simulink model "S_SSM"  (R2022b)
settings: Solver=VariableStepAuto  StartTime=0.0  StopTime=20  RelTol=1e-3
values from neighbouring files (symbols this model uses):
  Kd = place(Ad,Bd,p_discretos)    [Sist_ident.m]
  Kdl = place(A,B,pc)    [Sist_ident.m]
  wnc = 4.6/(tsc*zitac)    [Sist_ident.m]
  zitac = sqrt(((log(Mpc))^2)/(((log(Mpc))^2)+ pi^2))    [Sist_ident.m]
undefined symbols (not defined in the file or in its folder): Ad, Adl, Bd, Bdl, Cd, Cdl
libraries: slpidlib x1
settings Model: Creator=juand  LastModifiedBy=juand

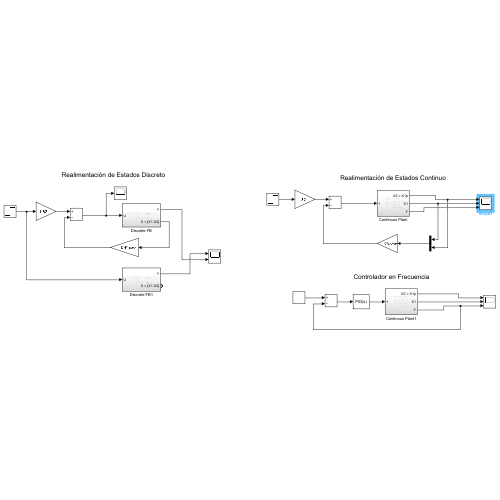
[thumbnail: Simulink's stored preview of the top-level diagram]
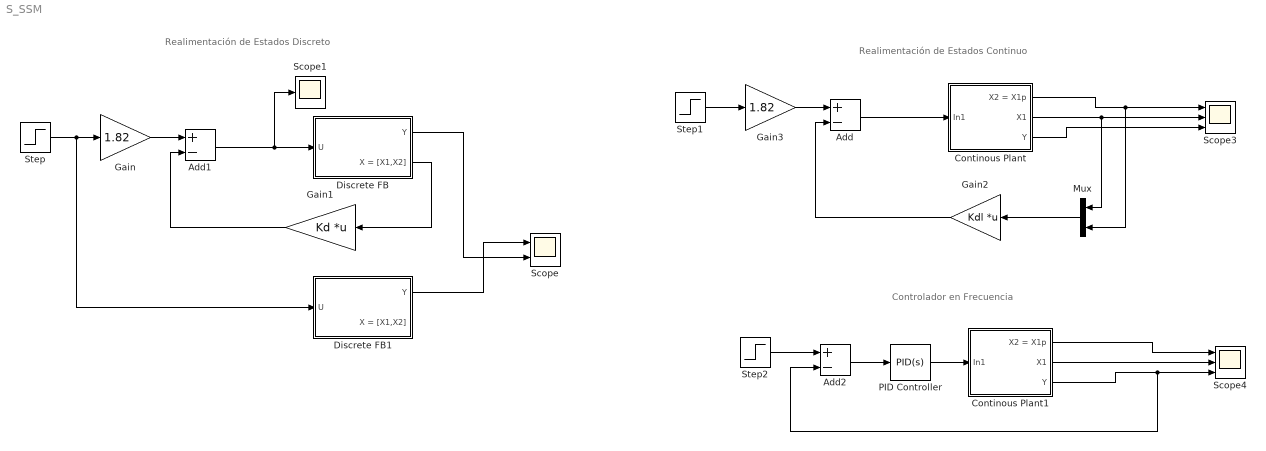
== system S_SSM ==
  note: Controlador en Frecuencia
  note: Realimentación de Estados Continuo
  note: Realimentación de Estados Discreto
  Add : Sum  Inputs=+-
  Add1 : Sum  Inputs=+-
  Add2 : Sum  Inputs=+-
  Continous Plant : Subsystem
  Continous Plant1 : Subsystem
  Discrete FB : Subsystem
  Discrete FB1 : Subsystem
  Gain : Gain  Gain=1.82
  Gain1 : Gain  Gain=Kd  Multiplication=Matrix(K*u) (u vector)
  Gain2 : Gain  Gain=Kdl  Multiplication=Matrix(K*u) (u vector)
  Gain3 : Gain  Gain=1.82
  Mux : Mux  Inputs=2
  PID Controller : slpidlib/PID Controller  Controller=PID  Form=Parallel  TimeDomain=Continuous-time  UseExternalTs=off  SampleTime=-1  IntegratorMethod=Forward Euler  FilterMethod=Forward Euler  ControllerParametersSource=internal  P=482.65  I=1036.21  UseKiTs=off  D=123.64  N=100  UseFilter=on  TunerSelectOption=Transfer Function Based (PID Tuner App)  InitialConditionSource=internal  InitialConditionForIntegrator=0  InitialConditionForFilter=0  DifferentiatorICPrevScaledInput=0  ExternalReset=none  TrackingMode=off  Kt=1  LimitOutput=off  SatLimitsSource=internal  UpperSaturationLimit=inf  LowerSaturationLimit=-inf  LinearizeAsGain=on  AntiWindupMode=none  Kb=1  LimitIntegrator=off  UpperIntegratorSaturationLimit=inf  LowerIntegratorSaturationLimit=-inf  POutMin=[]  POutMax=[]  IOutMin=[]  IOutMax=[]  DOutMin=[]  DOutMax=[]  NOutMin=[]  NOutMax=[]  SumOutMin=[]  SumOutMax=[]  SaturationOutMin=[]  SaturationOutMax=[]  PParamMin=[]  PParamMax=[]  IParamMin=[]  IParamMax=[]  DParamMin=[]  DParamMax=[]  NParamMin=[]  NParamMax=[]  KbParamMin=[]  KbParamMax=[]  KtParamMin=[]  KtParamMax=[]  KbOutMin=[]  KbOutMax=[]  KtOutMin=[]  KtOutMax=[]  IntegratorOutMin=[]  IntegratorOutMax=[]  FilterOutMin=[]  FilterOutMax=[]  SumI1OutMin=[]  SumI1OutMax=[]  SumI2OutMin=[]  SumI2OutMax=[]  SumI3OutMin=[]  SumI3OutMax=[]  SumI4OutMin=[]  SumI4OutMax=[]  SumDOutMin=[]  SumDOutMax=[]  DifferentiatorOutMin=[]  DifferentiatorOutMax=[]  FilterDiffOutCoefMin=[]  FilterDiffOutCoefMax=[]  ReciprocalOutMin=[]  ReciprocalOutMax=[]  SumDenOutMin=[]  SumDenOutMax=[]  SumNumOutMin=[]  SumNumOutMax=[]  DivideOutMin=[]  DivideOutMax=[]  UdiffTsProdOutMin=[]  UdiffTsProdOutMax=[]  NTsProdOutMin=[]  NTsProdOutMax=[]  UintegralTsProdOutMin=[]  UintegralTsProdOutMax=[]  UngainTsProdOutMin=[]  UngainTsProdOutMax=[]  ClampingZeroOutDataTypeStr=Inherit: Inherit via back propagation  ClampingZeroOutMin=[]  ClampingZeroOutMax=[]  FilterDenConstantOutDataTypeStr=Inherit: Inherit via back propagation  FilterDenConstantOutMin=[]  FilterDenConstantOutMax=[]  PCopyOutDataTypeStr=Inherit: Inherit via back propagation  PCopyOutMin=[]  PCopyOutMax=[]  NCopyOutDataTypeStr=Inherit: Inherit via back propagation  NCopyOutMin=[]  NCopyOutMax=[]  IntegratorContinuousStateAttributes=''  IntegratorStateMustResolveToSignalObject=off  IntegratorRTWStateStorageClass=Auto  FilterContinuousStateAttributes=''  FilterStateMustResolveToSignalObject=off  FilterRTWStateStorageClass=Auto  ParallelPVariant=InternalParameters  IdealPVariant=Disabled  IVariant=InternalParameters  DVariant=InternalParameters  IntegratorVariant=Continuous  SatVariant=Disabled  AWVariant=Passthrough  PCopyVariant=Disabled  TRVariant=Disabled  FdbkBlocksVariant=Forward  IdealPFdbkVariant=Disabled  SatFdbkVariant=Disabled  DerivativeFilterVariant=ContFilter  NVariant=InternalParameters  NCopyVariant=Disabled  FilterICVariant=InternalICsFilter  IntegratorICVariant=InternalICs  ExternalResetVariant=Disabled  TRSumVariant=Passthrough  SumFdbkVariant=Disabled  SumVariant=Sum_PID  TsampFilterVariant=InternalTs  TsampNgainVariant=Passthrough  TsampIntegralVariant=Passthrough  ExternalSaturationOutDataTypeStr=Inherit: Same as second input
  Scope : Scope  NumInputPorts=2
  Scope1 : Scope
  Scope3 : Scope  NumInputPorts=3
  Scope4 : Scope  NumInputPorts=3
  Step : Step  SampleTime=0.0488280999999979
  Step1 : Step  SampleTime=0
  Step2 : Step  SampleTime=0
  wires:
  Gain1/1 -> Add1/2
  Discrete FB/2(X = [X1,X2]) -> Gain1/1
  Add1/1 -> Scope1/1, Discrete FB/1(U)
  Step/1 -> Discrete FB1/1(U), Gain/1
  Gain/1 -> Add1/1
  Continous Plant/1(X2 = X1p) -> Mux/2, Scope3/1
  Continous Plant/2(X1) -> Mux/1, Scope3/2
  Continous Plant/3(Y) -> Scope3/3
  Mux/1 -> Gain2/1
  Add/1 -> Continous Plant/1(In1)
  Gain2/1 -> Add/2
  Continous Plant1/2(X1) -> Scope4/2
  Step2/1 -> Add2/1
  Continous Plant1/3(Y) -> Add2/2, Scope4/3
  Continous Plant1/1(X2 = X1p) -> Scope4/1
  Add2/1 -> PID Controller/1
  PID Controller/1 -> Continous Plant1/1(In1)
  Discrete FB1/1(Y) -> Scope/1
  Discrete FB/1(Y) -> Scope/2
  Gain3/1 -> Add/1
  Step1/1 -> Gain3/1

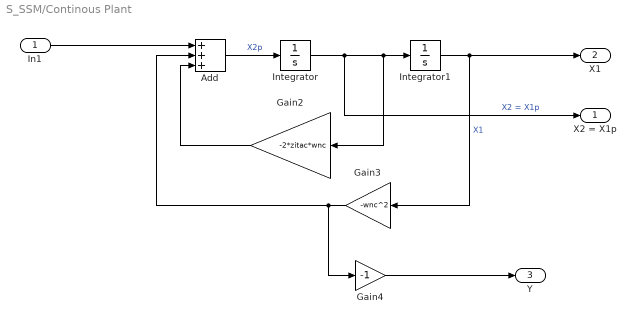
== system S_SSM/Continous Plant ==
  In1 : Inport
  Add : Sum  Inputs=+++
  Gain2 : Gain  Gain=-2*zitac*wnc
  Gain3 : Gain  Gain=-wnc^2
  Gain4 : Gain  Gain=-1
  Integrator : Integrator
  Integrator1 : Integrator
  X2 = X1p : Outport
  X1 : Outport  Port=2
  Y : Outport  Port=3
  wires:
  Integrator/1 -> X2 = X1p/1, Integrator1/1, Gain2/1  "X2 = X1p"
  Add/1 -> Integrator/1  "X2p"
  Integrator1/1 -> X1/1, Gain3/1  "X1"
  Gain3/1 -> Add/2, Gain4/1
  Gain4/1 -> Y/1
  In1/1 -> Add/1
  Gain2/1 -> Add/3

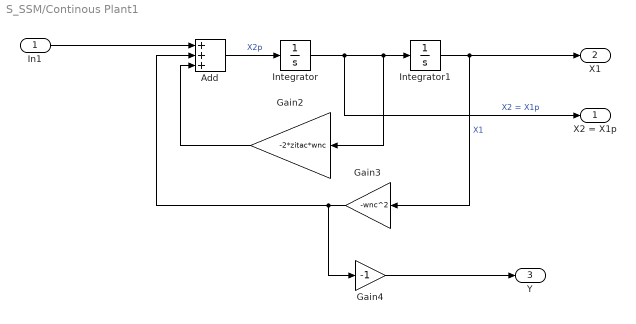
== system S_SSM/Continous Plant1 ==
  In1 : Inport
  Add : Sum  Inputs=+++
  Gain2 : Gain  Gain=-2*zitac*wnc
  Gain3 : Gain  Gain=-wnc^2
  Gain4 : Gain  Gain=-1
  Integrator : Integrator
  Integrator1 : Integrator
  X2 = X1p : Outport
  X1 : Outport  Port=2
  Y : Outport  Port=3
  wires:
  Integrator/1 -> X2 = X1p/1, Integrator1/1, Gain2/1  "X2 = X1p"
  Add/1 -> Integrator/1  "X2p"
  Integrator1/1 -> X1/1, Gain3/1  "X1"
  Gain3/1 -> Add/2, Gain4/1
  Gain4/1 -> Y/1
  In1/1 -> Add/1
  Gain2/1 -> Add/3

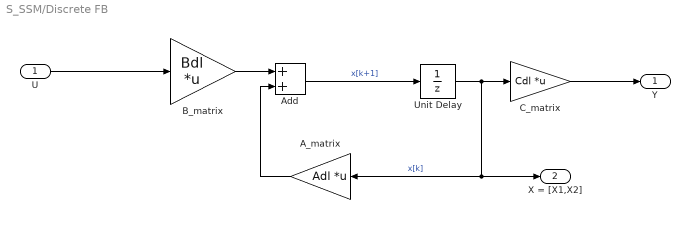
== system S_SSM/Discrete FB ==
  U : Inport
  A_matrix : Gain  Gain=Adl  Multiplication=Matrix(K*u) (u vector)
  Add : Sum
  B_matrix : Gain  Gain=Bdl  Multiplication=Matrix(K*u) (u vector)
  C_matrix : Gain  Gain=Cdl  Multiplication=Matrix(K*u) (u vector)
  Unit Delay : UnitDelay  SampleTime=0.0488280999999979  HasFrameUpgradeWarning=on
  Y : Outport
  X = [X1,X2] : Outport  Port=2
  wires:
  Add/1 -> Unit Delay/1  "x[k+1]"
  C_matrix/1 -> Y/1
  B_matrix/1 -> Add/1
  A_matrix/1 -> Add/2
  Unit Delay/1 -> A_matrix/1, X = [X1,X2]/1, C_matrix/1  "x[k]"
  U/1 -> B_matrix/1

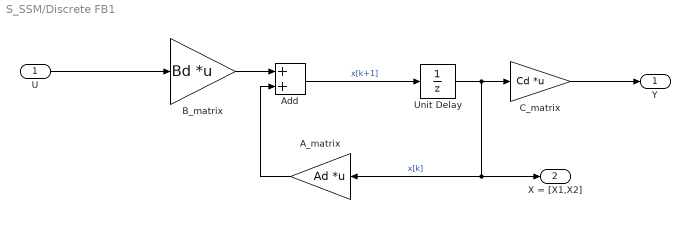
== system S_SSM/Discrete FB1 ==
  U : Inport
  A_matrix : Gain  Gain=Ad  Multiplication=Matrix(K*u) (u vector)
  Add : Sum
  B_matrix : Gain  Gain=Bd  Multiplication=Matrix(K*u) (u vector)
  C_matrix : Gain  Gain=Cd  Multiplication=Matrix(K*u) (u vector)
  Unit Delay : UnitDelay  SampleTime=0.0488280999999979  HasFrameUpgradeWarning=on
  Y : Outport
  X = [X1,X2] : Outport  Port=2
  wires:
  Add/1 -> Unit Delay/1  "x[k+1]"
  C_matrix/1 -> Y/1
  B_matrix/1 -> Add/1
  A_matrix/1 -> Add/2
  Unit Delay/1 -> A_matrix/1, X = [X1,X2]/1, C_matrix/1  "x[k]"
  U/1 -> B_matrix/1
